simulink model "Complete_Aircraft"  (R2020a)
settings: Solver=ode4  StartTime=0.0  StopTime=0  FixedStep=0.005  RelTol=1e-3
values from neighbouring files (symbols this model uses):
  b = 10.48    [parameters.m]    (also in poles.m; zeros_tf.m)
  beta_a = 9297    [parameters.m]    (also in poles.m; zeros_tf.m)
  cbar = 2.05    [parameters.m]
  CD0 = 0.023    [parameters.m]
  D = coeff(2)    [poles.m]
  da_trim = da_trim+dda    [parameters.m]
  de_trim = de_trim*(1+dde)    (= 0)    [parameters.m]
  df0 = 0+ddf    (= 0)    [parameters.m]
  dr_trim = dr_trim+ddr    [parameters.m]
  dth_trim = dth_trim*(1+ddt)    [parameters.m]
  E_ARM = [0 0 engine_arm]'    [parameters.m]
  grav = 9.81    [parameters.m]    (also in poles.m; zeros_tf.m)
  H0 = 3000    [parameters.m]    (also in poles.m; zeros_tf.m)
  Inertia = [Ixx   0   -Ixz ... (first row only)    [parameters.m]
  K = 1/pi/AR/e    (= 0.0734777604407)    [parameters.m]
  m = 0.7    [parameters.m]
  mass0 = mass_EO+mass_fuel+mass_res    (= 8000)    [parameters.m]
  mass_EO = 5000    [parameters.m]
  mass_res = 500    [parameters.m]
  MC_lat = [ Cy0 Cyb Cybdot Cyp Cyr Cyda Cydr ... (first row only)    [parameters.m]
  MC_lon = [ CL0 CLa CLadot CLq CLde CLdf ... (first row only)    [parameters.m]
  P0 = P0+dp    [parameters.m]    (also in poles.m = -0.0043; zeros_tf.m = -0.0043)
  Phi0 = Phi_i1    (= 0)    [parameters.m]    (also in poles.m = 0.705; zeros_tf.m = 0.705)
  Psi0 = 0    [parameters.m]
  Q0 = Q0+dq    [parameters.m]    (also in poles.m = 0.0338; zeros_tf.m = 0.0338)
  R0 = R0+dr    [parameters.m]    (also in poles.m = 0.0397; zeros_tf.m = 0.0397)
  rho_SL = 1.225    [parameters.m]    (also in poles.m; zeros_tf.m)
  S = 21.55    [parameters.m]    (also in poles.m; zeros_tf.m)
  sfc = (0.7)/3600    (= 0.000194444444444)    [parameters.m]
  T_TB = [cos(eps0) 0 sin(eps0) ... (first row only)    [parameters.m]
  Theta0 = (alpha_trim+gamma0)    [parameters.m]    (also in poles.m = 0.0827; zeros_tf.m = 0.0827)
  TmaxSL = 35000    [parameters.m]
  U0 = U0*(1+du)    [parameters.m]    (also in poles.m = 158.1484; zeros_tf.m = 158.1484)
  V0 = V0+dv    [parameters.m]
  W0 = W0*(1+dw)    [parameters.m]    (also in poles.m = 13.1075; zeros_tf.m = 13.1075)
  XN0 = 0    [parameters.m]
  YE0 = 0    [parameters.m]
libraries: shared6dof x1, aerolibtransform2 x1, vrlib x1, simulink x1, aerolibasang x1
settings Model: Creator=fabrizio  LastModifiedBy=fabrizio
settings DataIOCC: ReturnWorkspaceOutputs=off
settings DebuggingCC: ArithmeticOperatorsInVariantConditions=warning
settings SFSimCC: CustomCodeUndefinedFunction=UseInterfaceOnly

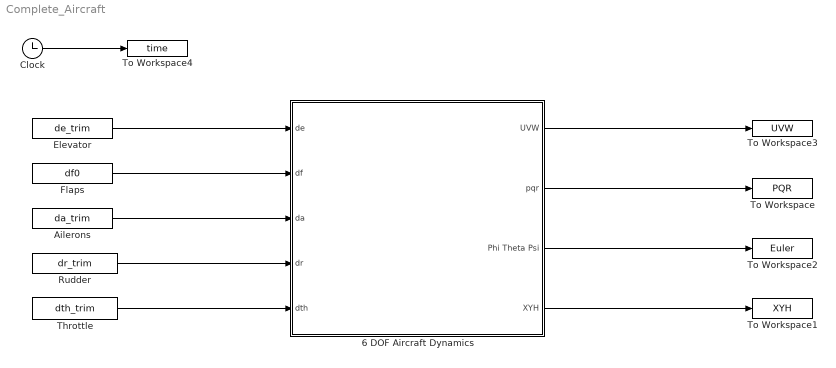
== system Complete_Aircraft ==
  6 DOF Aircraft Dynamics : Subsystem
  Ailerons : Constant  Value=da_trim
  Clock : Clock
  Elevator : Constant  Value=de_trim
  Flaps : Constant  Value=df0
  "Rudder " : Constant  Value=dr_trim
  "Throttle " : Constant  Value=dth_trim
  To Workspace : ToWorkspace  VariableName=PQR  SampleTime=-1
  To Workspace1 : ToWorkspace  VariableName=XYH  SampleTime=-1
  To Workspace2 : ToWorkspace  VariableName=Euler  SampleTime=-1
  To Workspace3 : ToWorkspace  VariableName=UVW  SampleTime=-1
  To Workspace4 : ToWorkspace  VariableName=time  SampleTime=-1
  wires:
  Elevator/1 -> 6 DOF Aircraft Dynamics/1(de)
  Flaps/1 -> 6 DOF Aircraft Dynamics/2(df)
  "Throttle "/1 -> 6 DOF Aircraft Dynamics/5(dth)
  "Rudder "/1 -> 6 DOF Aircraft Dynamics/4(dr)
  Ailerons/1 -> 6 DOF Aircraft Dynamics/3(da)
  6 DOF Aircraft Dynamics/1(UVW) -> To Workspace3/1
  6 DOF Aircraft Dynamics/2(pqr) -> To Workspace/1
  6 DOF Aircraft Dynamics/3(Phi Theta Psi) -> To Workspace2/1
  6 DOF Aircraft Dynamics/4(XYH) -> To Workspace1/1
  Clock/1 -> To Workspace4/1

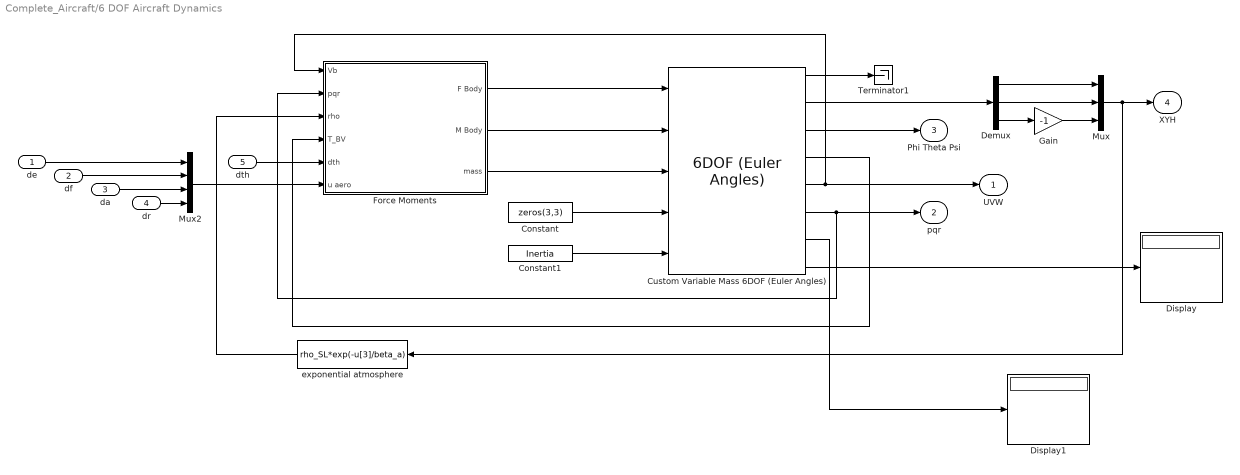
== system Complete_Aircraft/6 DOF Aircraft Dynamics ==
  de : Inport
  df : Inport  Port=2
  da : Inport  Port=3
  dr : Inport  Port=4
  dth : Inport  Port=5
  Constant : Constant  Value=zeros(3,3)
  Constant1 : Constant  Value=Inertia
  Custom Variable Mass 6DOF (Euler Angles) : shared6dof/6DOF (Euler Angles)  units=Metric (MKS)  mtype=Custom Variable  rep=Euler Angles  xme_0=[XN0 YE0 -H0]  Vm_0=[U0 V0 W0]  eul_0=[Phi0 Theta0 Psi0]  pm_0=[P0 Q0 R0]  mass_0=1.0  mass_e=0.5  mass_f=2.0  inertia=eye(3)  inertia_e=eye(3)  inertia_f=2*eye(3)  k_quat=1.0  vre_flag=off  abi_flag=off  aMode=0  xme_statename=''  Vm_statename=''  eul_statename=''  quat_statename=''  pm_statename=''  mass_statename=''
      settings: SourceProductBaseCode=AE,PW,MT,VE,VP
  Demux : Demux  Outputs=3
  Display : Display
  Display1 : Display
  Force Moments : Subsystem
  Gain : Gain  Gain=-1
  Mux : Mux  Inputs=3
  Mux2 : Mux
  Terminator1 : Terminator
  exponential atmosphere : Fcn  Expr=rho_SL*exp(-u[3]/beta_a)
  UVW : Outport  VectorParamsAs1DForOutWhenUnconnected=off
  pqr : Outport  Port=2  VectorParamsAs1DForOutWhenUnconnected=off
  Phi Theta Psi : Outport  Port=3  VectorParamsAs1DForOutWhenUnconnected=off
  XYH : Outport  Port=4  VectorParamsAs1DForOutWhenUnconnected=off
  wires:
  dr/1 -> Mux2/4
  df/1 -> Mux2/2
  dth/1 -> Force Moments/5(dth)
  exponential atmosphere/1 -> Force Moments/3(rho)
  da/1 -> Mux2/3
  de/1 -> Mux2/1
  Mux2/1 -> Force Moments/6(u aero)
  Force Moments/1(F Body) -> Custom Variable Mass 6DOF (Euler Angles)/1
  Force Moments/2(M Body) -> Custom Variable Mass 6DOF (Euler Angles)/2
  Force Moments/3(mass) -> Custom Variable Mass 6DOF (Euler Angles)/3
  Constant/1 -> Custom Variable Mass 6DOF (Euler Angles)/4
  Constant1/1 -> Custom Variable Mass 6DOF (Euler Angles)/5
  Custom Variable Mass 6DOF (Euler Angles)/8 -> Display/1
  Custom Variable Mass 6DOF (Euler Angles)/1 -> Terminator1/1
  Custom Variable Mass 6DOF (Euler Angles)/7 -> Display1/1
  Custom Variable Mass 6DOF (Euler Angles)/2 -> Demux/1
  Custom Variable Mass 6DOF (Euler Angles)/3 -> Phi Theta Psi/1
  Custom Variable Mass 6DOF (Euler Angles)/5 -> Force Moments/1(Vb), UVW/1
  Custom Variable Mass 6DOF (Euler Angles)/6 -> Force Moments/2(pqr), pqr/1
  Custom Variable Mass 6DOF (Euler Angles)/4 -> Force Moments/4(T_BV)
  Demux/1 -> Mux/1
  Demux/2 -> Mux/2
  Demux/3 -> Gain/1
  Gain/1 -> Mux/3
  Mux/1 -> XYH/1, exponential atmosphere/1

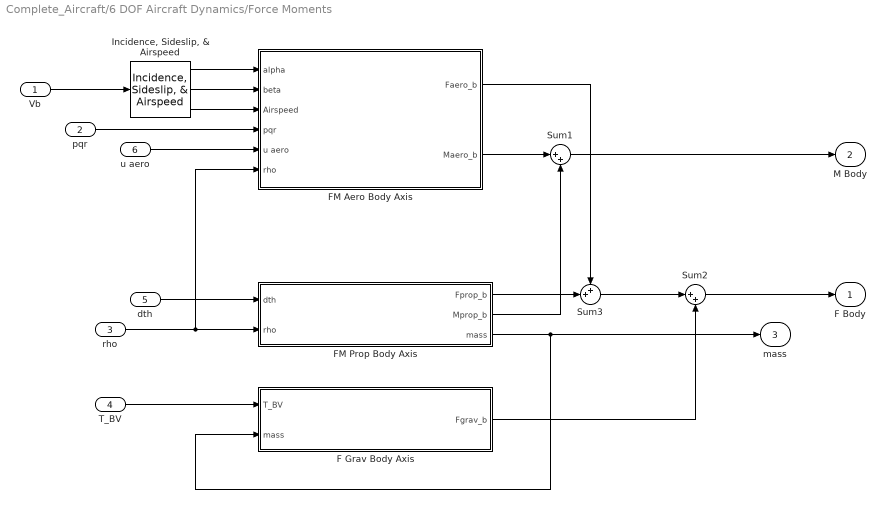
== system Complete_Aircraft/6 DOF Aircraft Dynamics/Force Moments ==
  Vb : Inport
  pqr : Inport  Port=2
  rho : Inport  Port=3
  T_BV : Inport  Port=4
  dth : Inport  Port=5
  u aero : Inport  Port=6
  F Grav Body Axis : Subsystem
  FM Aero Body Axis : Subsystem
  FM Prop Body Axis : Subsystem
  "Incidence, Sideslip, & Airspeed" : aerolibasang/Incidence, Sideslip, & Airspeed
  Sum1 : Sum  Inputs=|++
  Sum2 : Sum  Inputs=|++
  Sum3 : Sum  Inputs=++|
  F Body : Outport  VectorParamsAs1DForOutWhenUnconnected=off
  M Body : Outport  Port=2  VectorParamsAs1DForOutWhenUnconnected=off
  mass : Outport  Port=3  VectorParamsAs1DForOutWhenUnconnected=off
  wires:
  dth/1 -> FM Prop Body Axis/1(dth)
  pqr/1 -> FM Aero Body Axis/4(pqr)
  FM Prop Body Axis/2(Mprop_b) -> Sum1/2
  rho/1 -> FM Aero Body Axis/6(rho), FM Prop Body Axis/2(rho)
  FM Aero Body Axis/2(Maero_b) -> Sum1/1
  "Incidence, Sideslip, & Airspeed"/3 -> FM Aero Body Axis/3(Airspeed)
  "Incidence, Sideslip, & Airspeed"/1 -> FM Aero Body Axis/1(alpha)
  "Incidence, Sideslip, & Airspeed"/2 -> FM Aero Body Axis/2(beta)
  T_BV/1 -> F Grav Body Axis/1(T_BV)
  Sum1/1 -> M Body/1
  FM Prop Body Axis/3(mass) -> mass/1, F Grav Body Axis/2(mass)
  Vb/1 -> "Incidence, Sideslip, & Airspeed"/1
  u aero/1 -> FM Aero Body Axis/5(u aero)
  Sum3/1 -> Sum2/1
  FM Prop Body Axis/1(Fprop_b) -> Sum3/2
  FM Aero Body Axis/1(Faero_b) -> Sum3/1
  F Grav Body Axis/1(Fgrav_b) -> Sum2/2
  Sum2/1 -> F Body/1

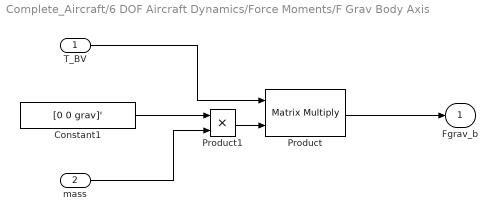
== system Complete_Aircraft/6 DOF Aircraft Dynamics/Force Moments/F Grav Body Axis ==
  T_BV : Inport
  mass : Inport  Port=2
  Constant1 : Constant  Value=[0 0 grav]'
  Product : Product  Multiplication=Matrix(*)
  Product1 : Product
  Fgrav_b : Outport  VectorParamsAs1DForOutWhenUnconnected=off
  wires:
  Product/1 -> Fgrav_b/1
  T_BV/1 -> Product/1
  Constant1/1 -> Product1/1
  Product1/1 -> Product/2
  mass/1 -> Product1/2

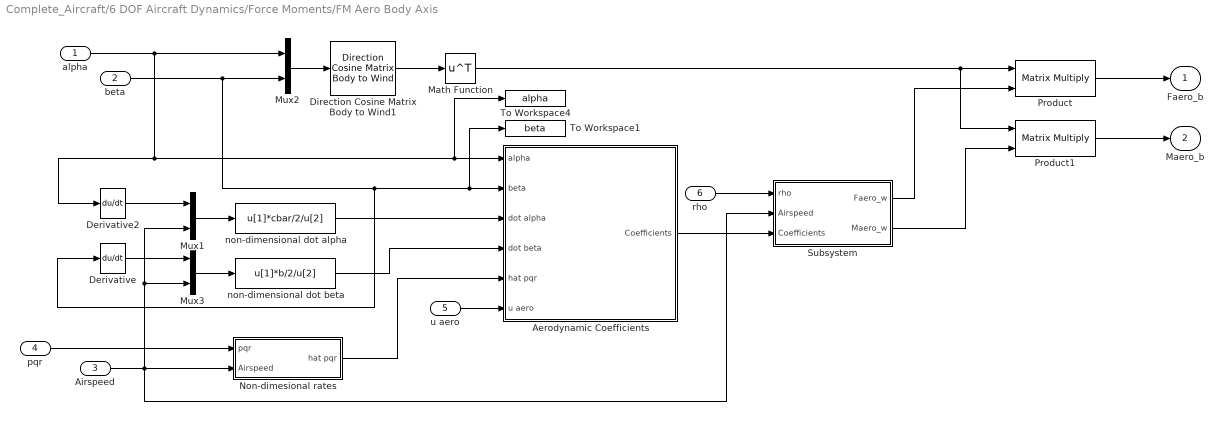
== system Complete_Aircraft/6 DOF Aircraft Dynamics/Force Moments/FM Aero Body Axis ==
  alpha : Inport
  beta : Inport  Port=2
  Airspeed : Inport  Port=3
  pqr : Inport  Port=4
  u aero : Inport  Port=5
  rho : Inport  Port=6
  Aerodynamic Coefficients : Subsystem
  Derivative : Derivative
  Derivative2 : Derivative
  Direction Cosine Matrix Body to Wind1 : aerolibtransform2/Direction Cosine Matrix Body to Wind
      settings: SourceProductBaseCode=AE
  Math Function : Math  Operator=transpose  SignedPower=on  SaturateOnIntegerOverflow=on
  Mux1 : Mux  Inputs=2
  Mux2 : Mux  Inputs=2
  Mux3 : Mux  Inputs=2
  Non-dimesional rates : Subsystem
  Product : Product  Multiplication=Matrix(*)
  Product1 : Product  Multiplication=Matrix(*)
  Subsystem : Subsystem
  To Workspace1 : ToWorkspace  VariableName=beta  SampleTime=-1
  To Workspace4 : ToWorkspace  VariableName=alpha  SampleTime=-1
  non-dimensional dot alpha : Fcn  Expr=u[1]*cbar/2/u[2]
  "non-dimensional dot beta " : Fcn  Expr=u[1]*b/2/u[2]
  Faero_b : Outport  VectorParamsAs1DForOutWhenUnconnected=off
  Maero_b : Outport  Port=2  VectorParamsAs1DForOutWhenUnconnected=off
  wires:
  rho/1 -> Subsystem/1(rho)
  pqr/1 -> Non-dimesional rates/1(pqr)
  Non-dimesional rates/1(hat pqr) -> Aerodynamic Coefficients/5(hat pqr)
  Aerodynamic Coefficients/1(Coefficients) -> Subsystem/3(Coefficients)
  Airspeed/1 -> Subsystem/2(Airspeed), Mux1/2, Mux3/2, Non-dimesional rates/2(Airspeed)
  Math Function/1 -> Product1/1, Product/1
  Direction Cosine Matrix Body to Wind1/1 -> Math Function/1
  Mux2/1 -> Direction Cosine Matrix Body to Wind1/1
  Product/1 -> Faero_b/1
  Product1/1 -> Maero_b/1
  Subsystem/1(Faero_w) -> Product/2
  Subsystem/2(Maero_w) -> Product1/2
  u aero/1 -> Aerodynamic Coefficients/6(u aero)
  alpha/1 -> Mux2/1, Derivative2/1, To Workspace4/1, Aerodynamic Coefficients/1(alpha)
  beta/1 -> Derivative/1, To Workspace1/1, Aerodynamic Coefficients/2(beta), Mux2/2
  Mux3/1 -> "non-dimensional dot beta "/1
  Derivative/1 -> Mux3/1
  Derivative2/1 -> Mux1/1
  Mux1/1 -> non-dimensional dot alpha/1
  non-dimensional dot alpha/1 -> Aerodynamic Coefficients/3(dot alpha)
  "non-dimensional dot beta "/1 -> Aerodynamic Coefficients/4(dot beta)

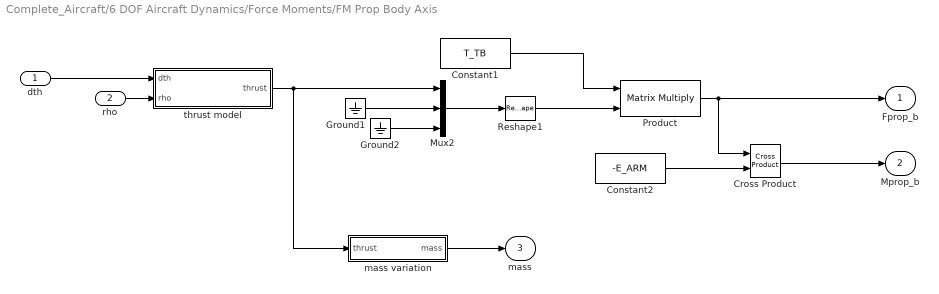
== system Complete_Aircraft/6 DOF Aircraft Dynamics/Force Moments/FM Prop Body Axis ==
  dth : Inport
  rho : Inport  Port=2
  Constant1 : Constant  Value=T_TB
  Constant2 : Constant  Value=-E_ARM
  Cross Product : vrlib/Utilities/Cross Product
  Ground1 : Ground
  Ground2 : Ground
  Mux2 : Mux  Inputs=3
  Product : Product  Multiplication=Matrix(*)
  Reshape1 : Reshape  OutputDimensionality=Column vector (2-D)
  mass variation : Subsystem
  thrust model : Subsystem
  Fprop_b : Outport  VectorParamsAs1DForOutWhenUnconnected=off
  Mprop_b : Outport  Port=2  VectorParamsAs1DForOutWhenUnconnected=off
  mass : Outport  Port=3  VectorParamsAs1DForOutWhenUnconnected=off
  wires:
  Constant1/1 -> Product/1
  Cross Product/1 -> Mprop_b/1
  Constant2/1 -> Cross Product/2
  Mux2/1 -> Reshape1/1
  Ground2/1 -> Mux2/3
  rho/1 -> thrust model/2(rho)
  Ground1/1 -> Mux2/2
  thrust model/1("thrust ") -> mass variation/1(thrust), Mux2/1
  Product/1 -> Fprop_b/1, Cross Product/1
  dth/1 -> thrust model/1(dth)
  mass variation/1("mass ") -> mass/1
  Reshape1/1 -> Product/2

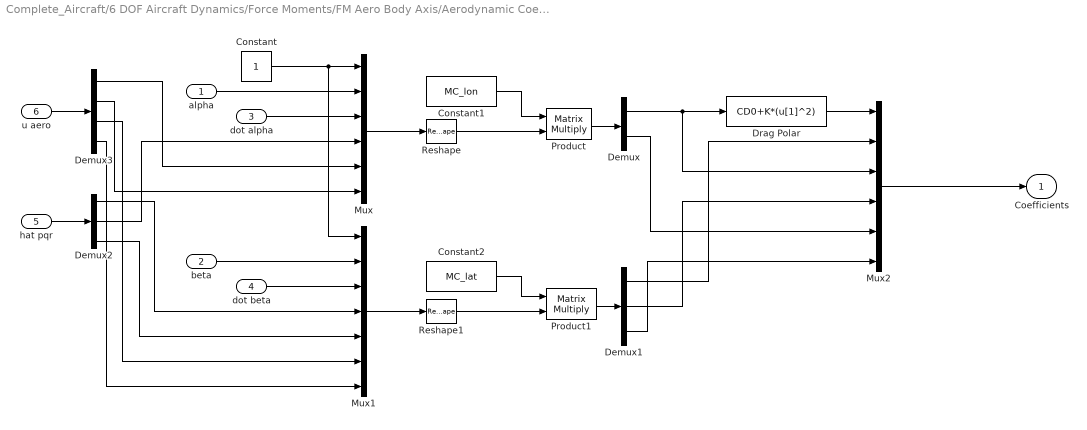
== system Complete_Aircraft/6 DOF Aircraft Dynamics/Force Moments/FM Aero Body Axis/Aerodynamic Coefficients ==
  alpha : Inport
  beta : Inport  Port=2
  dot alpha : Inport  Port=3
  dot beta : Inport  Port=4
  hat pqr : Inport  Port=5
  u aero : Inport  Port=6
  Constant : Constant
  Constant1 : Constant  Value=MC_lon
  Constant2 : Constant  Value=MC_lat
  Demux : Demux  Outputs=2
  Demux1 : Demux  Outputs=[1 1 1]
  Demux2 : Demux  Outputs=3
  Demux3 : Demux
  Drag Polar : Fcn  Expr=CD0+K*(u[1]^2)
  Mux : Mux  Inputs=6
  Mux1 : Mux  Inputs=7
  Mux2 : Mux  Inputs=6
  Product : Product  Multiplication=Matrix(*)
  Product1 : Product  Multiplication=Matrix(*)
  Reshape : Reshape  OutputDimensionality=Column vector (2-D)
  Reshape1 : Reshape  OutputDimensionality=Column vector (2-D)
  Coefficients : Outport  VectorParamsAs1DForOutWhenUnconnected=off
  wires:
  Constant1/1 -> Product/1
  Product/1 -> Demux/1
  dot alpha/1 -> Mux/3
  Demux/1 -> Mux2/3, Drag Polar/1
  Demux/2 -> Mux2/5
  Constant2/1 -> Product1/1
  Product1/1 -> Demux1/1
  Demux3/1 -> Mux/5
  beta/1 -> Mux1/2
  Demux1/2 -> Mux2/4
  Constant/1 -> Mux1/1, Mux/1
  Demux3/2 -> Mux/6
  Drag Polar/1 -> Mux2/1
  Demux1/1 -> Mux2/2
  Mux/1 -> Reshape/1
  dot beta/1 -> Mux1/3
  Mux1/1 -> Reshape1/1
  Demux3/4 -> Mux1/7
  alpha/1 -> Mux/2
  Demux1/3 -> Mux2/6
  Mux2/1 -> Coefficients/1
  hat pqr/1 -> Demux2/1
  Demux2/2 -> Mux/4
  Demux2/1 -> Mux1/4
  Demux2/3 -> Mux1/5
  Demux3/3 -> Mux1/6
  u aero/1 -> Demux3/1
  Reshape/1 -> Product/2
  Reshape1/1 -> Product1/2

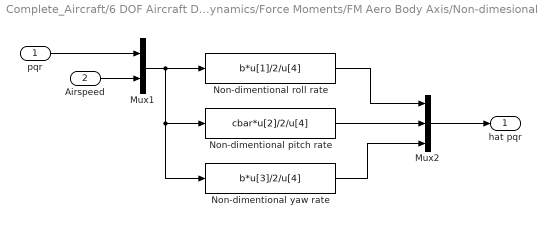
== system Complete_Aircraft/6 DOF Aircraft Dynamics/Force Moments/FM Aero Body Axis/Non-dimesional rates ==
  pqr : Inport
  Airspeed : Inport  Port=2
  Mux1 : Mux  Inputs=[3 1]
  Mux2 : Mux  Inputs=3
  Non-dimentional pitch rate : Fcn  Expr=cbar*u[2]/2/u[4]
  Non-dimentional roll rate : Fcn  Expr=b*u[1]/2/u[4]
  Non-dimentional yaw rate : Fcn  Expr=b*u[3]/2/u[4]
  hat pqr : Outport  VectorParamsAs1DForOutWhenUnconnected=off
  wires:
  pqr/1 -> Mux1/1
  Airspeed/1 -> Mux1/2
  Non-dimentional yaw rate/1 -> Mux2/3
  Mux1/1 -> Non-dimentional yaw rate/1, Non-dimentional pitch rate/1, Non-dimentional roll rate/1
  Mux2/1 -> hat pqr/1
  Non-dimentional pitch rate/1 -> Mux2/2
  Non-dimentional roll rate/1 -> Mux2/1

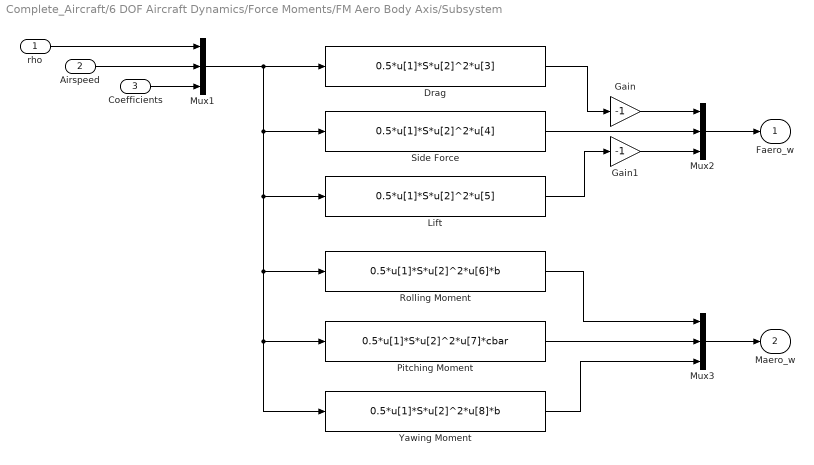
== system Complete_Aircraft/6 DOF Aircraft Dynamics/Force Moments/FM Aero Body Axis/Subsystem ==
  rho : Inport
  Airspeed : Inport  Port=2
  Coefficients : Inport  Port=3
  Drag : Fcn  Expr=0.5*u[1]*S*u[2]^2*u[3]
  Gain : Gain  Gain=-1
  Gain1 : Gain  Gain=-1
  "Lift " : Fcn  Expr=0.5*u[1]*S*u[2]^2*u[5]
  Mux1 : Mux  Inputs=[1 1 6]
  Mux2 : Mux  Inputs=3
  Mux3 : Mux  Inputs=3
  Pitching Moment : Fcn  Expr=0.5*u[1]*S*u[2]^2*u[7]*cbar
  Rolling Moment : Fcn  Expr=0.5*u[1]*S*u[2]^2*u[6]*b
  Side Force : Fcn  Expr=0.5*u[1]*S*u[2]^2*u[4]
  Yawing Moment : Fcn  Expr=0.5*u[1]*S*u[2]^2*u[8]*b
  Faero_w : Outport  VectorParamsAs1DForOutWhenUnconnected=off
  Maero_w : Outport  Port=2  VectorParamsAs1DForOutWhenUnconnected=off
  wires:
  Airspeed/1 -> Mux1/2
  rho/1 -> Mux1/1
  Mux1/1 -> Yawing Moment/1, Pitching Moment/1, Rolling Moment/1, "Lift "/1, Side Force/1, Drag/1
  Coefficients/1 -> Mux1/3
  Side Force/1 -> Mux2/2
  "Lift "/1 -> Gain1/1
  Drag/1 -> Gain/1
  Gain/1 -> Mux2/1
  Gain1/1 -> Mux2/3
  Pitching Moment/1 -> Mux3/2
  Yawing Moment/1 -> Mux3/3
  Rolling Moment/1 -> Mux3/1
  Mux2/1 -> Faero_w/1
  Mux3/1 -> Maero_w/1

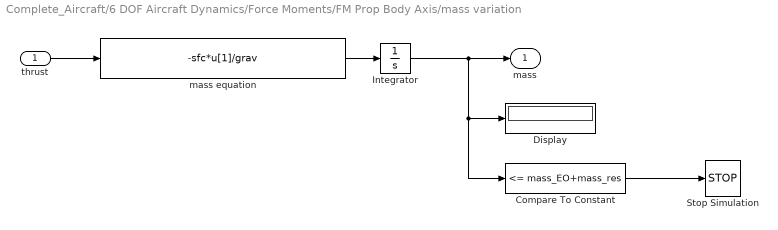
== system Complete_Aircraft/6 DOF Aircraft Dynamics/Force Moments/FM Prop Body Axis/mass variation ==
  thrust : Inport
  Compare To Constant : simulink/Logic and Bit Operations/Compare To Constant  relop=<=  const=mass_EO+mass_res  OutDataTypeStr=boolean
  Display : Display
  Integrator : Integrator  InitialCondition=mass0
  Stop Simulation : Stop
  mass equation : Fcn  Expr=-sfc*u[1]/grav
  "mass " : Outport  VectorParamsAs1DForOutWhenUnconnected=off
  wires:
  mass equation/1 -> Integrator/1
  Integrator/1 -> Compare To Constant/1, Display/1, "mass "/1
  thrust/1 -> mass equation/1
  Compare To Constant/1 -> Stop Simulation/1

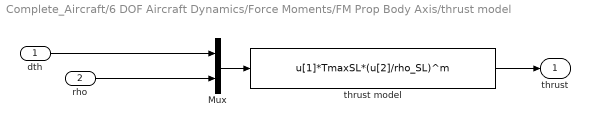
== system Complete_Aircraft/6 DOF Aircraft Dynamics/Force Moments/FM Prop Body Axis/thrust model ==
  dth : Inport
  rho : Inport  Port=2
  Mux : Mux  Inputs=2
  thrust model : Fcn  Expr=u[1]*TmaxSL*(u[2]/rho_SL)^m
  "thrust " : Outport  VectorParamsAs1DForOutWhenUnconnected=off
  wires:
  thrust model/1 -> "thrust "/1
  Mux/1 -> thrust model/1
  dth/1 -> Mux/1
  rho/1 -> Mux/2
